simulink model "Derating_Functions"  (R2024a)
settings: Solver=VariableStepAuto  StartTime=0.0  StopTime=10.0  RelTol=1e-3
libraries: simulink x3
settings Model: Creator=ezeki  LastModifiedBy=ezeki

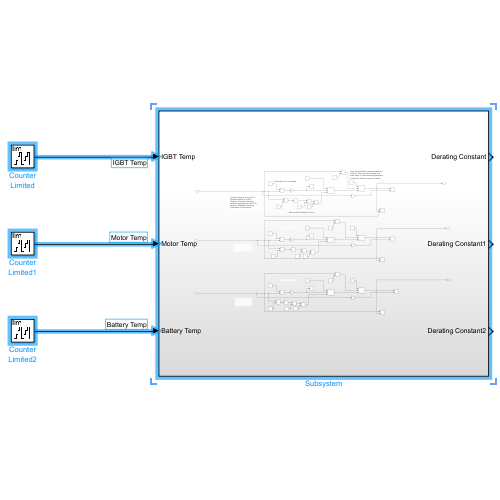
[thumbnail: Simulink's stored preview of the top-level diagram]
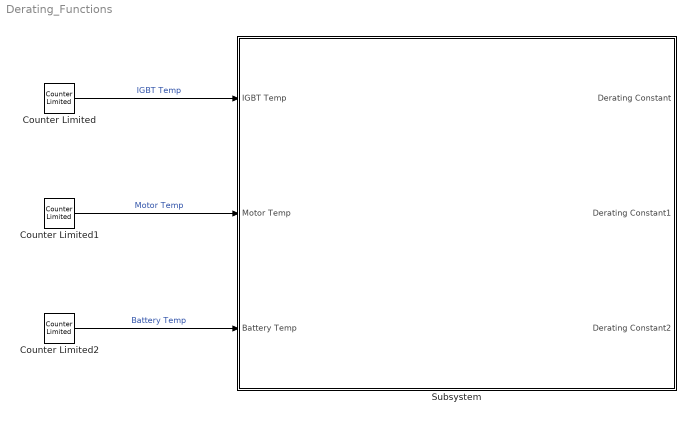
== system Derating_Functions ==
  Counter Limited : simulink/Sources/Counter Limited  uplimit=100  tsamp=0.1
  Counter Limited1 : simulink/Sources/Counter Limited  uplimit=150  tsamp=0.07
  Counter Limited2 : simulink/Sources/Counter Limited  uplimit=100  tsamp=0.1
  Subsystem : Subsystem
  wires:
  Counter Limited/1 -> Subsystem/1(IGBT Temp)  "IGBT Temp"
  Counter Limited1/1 -> Subsystem/2(Motor Temp)  "Motor Temp"
  Counter Limited2/1 -> Subsystem/3(Battery Temp)  "Battery Temp"

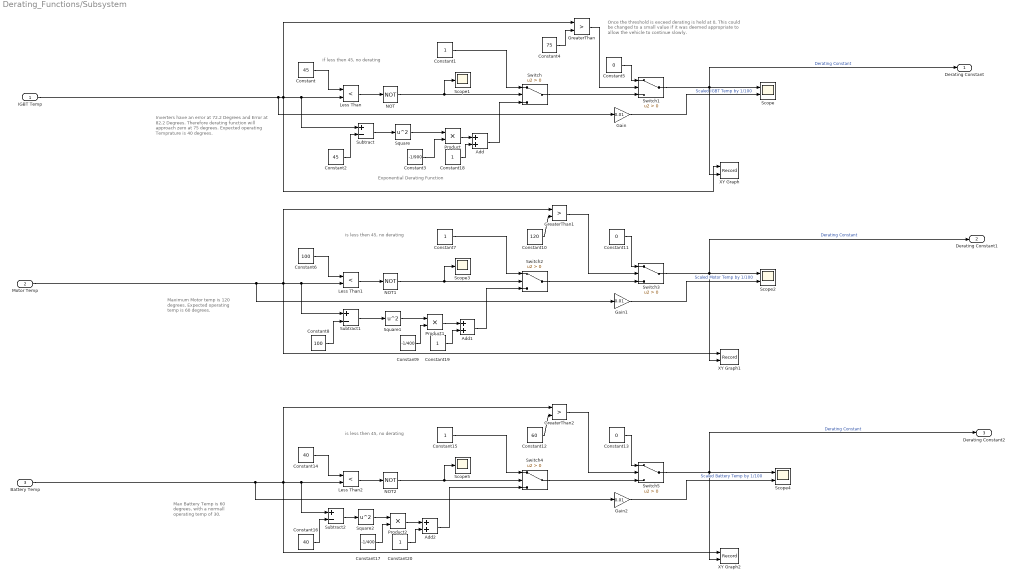
== system Derating_Functions/Subsystem ==
  note: Once the threshold is exceed derating is held at 0, This could be changed to a small value if it was deemed appropriate to allow the vehicle to continue slowly.
  note: Exponential Derating Function
  note: if less then 45, no derating
  note: Max Battery Temp is 60 degrees, with a normall operating temp of 30.
  note: Maximum Motor temp is 120 degrees. Expected operating temp is 60 degrees.
  note: Inverters have an error at 72.2 Degrees and Error at 82.2 Degrees. Therefore derating function will approach zero at 75 degrees. Expected operating Temprature is 40 degrees.
  note: is less then 45, no derating
  note: is less then 45, no derating
  IGBT Temp : Inport
  Motor Temp : Inport  Port=2
  Battery Temp : Inport  Port=3
  Add : Sum
  Add1 : Sum
  Add2 : Sum
  Constant : Constant  Value=45
  Constant{1,7,15,18..20} (6 alike) : Constant
  Constant10 : Constant  Value=120
  Constant11 : Constant  Value=0
  Constant12 : Constant  Value=60
  Constant13 : Constant  Value=0
  Constant14 : Constant  Value=40
  Constant16 : Constant  Value=40
  Constant17 : Constant  Value=-1/400
  Constant2 : Constant  Value=45
  Constant3 : Constant  Value=-1/900
  Constant4 : Constant  Value=75
  Constant5 : Constant  Value=0
  Constant6 : Constant  Value=100
  Constant8 : Constant  Value=100
  Constant9 : Constant  Value=-1/400
  Gain : Gain  Gain=0.01
  Gain1 : Gain  Gain=0.01
  Gain2 : Gain  Gain=0.01
  GreaterThan : RelationalOperator  Operator=>  OutDataTypeStr=boolean  RndMeth=Simplest  InputSameDT=off
  GreaterThan1 : RelationalOperator  Operator=>  OutDataTypeStr=boolean  RndMeth=Simplest  InputSameDT=off
  GreaterThan2 : RelationalOperator  Operator=>  OutDataTypeStr=boolean  RndMeth=Simplest  InputSameDT=off
  Less Than : RelationalOperator  Operator=<  OutDataTypeStr=boolean  RndMeth=Simplest  InputSameDT=off
  Less Than1 : RelationalOperator  Operator=<  OutDataTypeStr=boolean  RndMeth=Simplest  InputSameDT=off
  Less Than2 : RelationalOperator  Operator=<  OutDataTypeStr=boolean  RndMeth=Simplest  InputSameDT=off
  NOT : Logic  Operator=NOT  IconShape=distinctive  AllPortsSameDT=off  OutDataTypeStr=boolean
  NOT1 : Logic  Operator=NOT  IconShape=distinctive  AllPortsSameDT=off  OutDataTypeStr=boolean
  NOT2 : Logic  Operator=NOT  IconShape=distinctive  AllPortsSameDT=off  OutDataTypeStr=boolean
  Product : Product
  Product1 : Product
  Product2 : Product
  Scope : Scope  NumInputPorts=2
  Scope1 : Scope
  Scope2 : Scope  NumInputPorts=2
  Scope3 : Scope
  Scope4 : Scope  NumInputPorts=2
  Scope5 : Scope
  Square : Math  Operator=square
  Square1 : Math  Operator=square
  Square2 : Math  Operator=square
  Subtract : Sum  Inputs=+-
  Subtract1 : Sum  Inputs=+-
  Subtract2 : Sum  Inputs=+-
  Switch{,1..5} (6 alike) : Switch  Criteria=u2 > Threshold  SaturateOnIntegerOverflow=off  InputSameDT=off
  XY Graph : Record  FileSettingsInternal="{\"entries\":[{\"content\":{\"excelSettings\":{\"content\":{},\"type\":\"Streamout.ExcelSettings\"}},\"type\":\"Streamout.FileSettingStorage\",\"uuid\":\"\"}],\"packageUris\":[\"http:\\/\\/schema.mathworks.com\\/mf0\\/streamout_blocks\\/R2020a\"],\"version\":\"1.0\"}"  Layout=[1 1]  SignalsInternal="{\"entries\":[{\"content\":{\"signals\":[{\"content\":{\"blockPath\":[],\"dimensions\":[1],\"domain\":\"\",\"lineColor\":\"#a2142f\",\"plots\":[ 1 ],\"port\":1,\"signalID\":1,\"signalName\":\"IGBT Temp\"},\"type\":\"RecordBlkView.Signal\",\"uuid\":\"\"},{\"content\":{\"blockPath\":[],\"dimensions\":[1],\"domain\":\"\",\"lineColor\":\"#139fff\",\"plots\":[ 1 ],\"port\":2,\"signalID\":2,\"signalName\":\"Derating Constant\"},\"type\":\"RecordBlkView.Signal\",\"uuid\":\"\"}]},\"type\":\"RecordBlkView.InputSignals\",\"uuid\":\"\"}],\"packageUris\":[\"http:\\/\\/schema.mathworks.com\\/mf0\\/streamout_blocks\\/R2020a\"],\"version\":\"1.0\"}"  VisualizationBindings="{\"xyplotplugin\":{\"info\":[{\"series\":[{\"bindingParametersList\":[{\"parameter\":\"X-Axis\",\"signalID\":1,\"signalName\":\"IGBT Temp\"},{\"parameter\":\"Y-Axis\",\"signalID\":2,\"signalName\":\"Derating Constant\"}],\"seriesID\":0}],\"subplotID\":1}]}}"  CompatibilityTag=XY
  XY Graph1 : Record  FileSettingsInternal="{\"entries\":[{\"content\":{\"excelSettings\":{\"content\":{},\"type\":\"Streamout.ExcelSettings\"}},\"type\":\"Streamout.FileSettingStorage\",\"uuid\":\"\"}],\"packageUris\":[\"http:\\/\\/schema.mathworks.com\\/mf0\\/streamout_blocks\\/R2020a\"],\"version\":\"1.0\"}"  Layout=[1 1]  SignalsInternal="{\"entries\":[{\"content\":{\"signals\":[{\"content\":{\"blockPath\":[],\"dimensions\":[1],\"domain\":\"\",\"lineColor\":\"#a2142f\",\"plots\":[ 1 ],\"port\":1,\"signalID\":1,\"signalName\":\"Motor Temp\"},\"type\":\"RecordBlkView.Signal\",\"uuid\":\"\"},{\"content\":{\"blockPath\":[],\"dimensions\":[1],\"domain\":\"\",\"lineColor\":\"#139fff\",\"plots\":[ 1 ],\"port\":2,\"signalID\":2,\"signalName\":\"Derating Constant\"},\"type\":\"RecordBlkView.Signal\",\"uuid\":\"\"}]},\"type\":\"RecordBlkView.InputSignals\",\"uuid\":\"\"}],\"packageUris\":[\"http:\\/\\/schema.mathworks.com\\/mf0\\/streamout_blocks\\/R2020a\"],\"version\":\"1.0\"}"  VisualizationBindings="{\"xyplotplugin\":{\"info\":[{\"series\":[{\"bindingParametersList\":[{\"parameter\":\"X-Axis\",\"signalID\":1,\"signalName\":\"Motor Temp\"},{\"parameter\":\"Y-Axis\",\"signalID\":2,\"signalName\":\"Derating Constant\"}],\"seriesID\":0}],\"subplotID\":1}]}}"  CompatibilityTag=XY
  XY Graph2 : Record  FileSettingsInternal="{\"entries\":[{\"content\":{\"excelSettings\":{\"content\":{},\"type\":\"Streamout.ExcelSettings\"}},\"type\":\"Streamout.FileSettingStorage\",\"uuid\":\"\"}],\"packageUris\":[\"http:\\/\\/schema.mathworks.com\\/mf0\\/streamout_blocks\\/R2020a\"],\"version\":\"1.0\"}"  Layout=[1 1]  SignalsInternal="{\"entries\":[{\"content\":{\"signals\":[{\"content\":{\"blockPath\":[],\"dimensions\":[1],\"domain\":\"\",\"lineColor\":\"#a2142f\",\"plots\":[ 1 ],\"port\":1,\"signalID\":1,\"signalName\":\"Battery Temp\"},\"type\":\"RecordBlkView.Signal\",\"uuid\":\"\"},{\"content\":{\"blockPath\":[],\"dimensions\":[1],\"domain\":\"\",\"lineColor\":\"#139fff\",\"plots\":[ 1 ],\"port\":2,\"signalID\":2,\"signalName\":\"Derating Constant\"},\"type\":\"RecordBlkView.Signal\",\"uuid\":\"\"}]},\"type\":\"RecordBlkView.InputSignals\",\"uuid\":\"\"}],\"packageUris\":[\"http:\\/\\/schema.mathworks.com\\/mf0\\/streamout_blocks\\/R2020a\"],\"version\":\"1.0\"}"  VisualizationBindings="{\"xyplotplugin\":{\"info\":[{\"series\":[{\"bindingParametersList\":[{\"parameter\":\"X-Axis\",\"signalID\":1,\"signalName\":\"Battery Temp\"},{\"parameter\":\"Y-Axis\",\"signalID\":2,\"signalName\":\"Derating Constant\"}],\"seriesID\":0}],\"subplotID\":1}]}}"  CompatibilityTag=XY
  Derating Constant : Outport
  Derating Constant1 : Outport  Port=2
  Derating Constant2 : Outport  Port=3
  wires:
  Add/1 -> Switch/3
  Less Than2/1 -> NOT2/1
  Motor Temp/1 -> XY Graph1/1, GreaterThan1/1, Subtract1/1, Less Than1/2, Gain1/1
  NOT2/1 -> Scope5/1, Switch4/2
  Constant7/1 -> Switch2/1
  Switch1/1 -> Derating Constant/1, Scope/1, XY Graph/2  "Derating Constant"
  Gain1/1 -> Scope2/2  "Scaled Motor Temp by 1/100"
  NOT1/1 -> Scope3/1, Switch2/2
  GreaterThan/1 -> Switch1/2
  Constant18/1 -> Add/2
  Constant16/1 -> Subtract2/2
  Subtract1/1 -> Square1/1
  Constant1/1 -> Switch/1
  Battery Temp/1 -> XY Graph2/1, GreaterThan2/1, Subtract2/1, Less Than2/2, Gain2/1
  Subtract2/1 -> Square2/1
  Constant5/1 -> Switch1/1
  Switch/1 -> Switch1/3
  Less Than/1 -> NOT/1
  Product1/1 -> Add1/1
  Constant2/1 -> Subtract/2
  Constant6/1 -> Less Than1/1
  Subtract/1 -> Square/1
  Gain2/1 -> Scope4/2  "Scaled Battery Temp by 1/100"
  Add1/1 -> Switch2/3
  Add2/1 -> Switch4/3
  Constant19/1 -> Add1/2
  Constant8/1 -> Subtract1/2
  Square/1 -> Product/1
  Constant9/1 -> Product1/2
  Constant4/1 -> GreaterThan/2
  IGBT Temp/1 -> Gain/1, XY Graph/1, GreaterThan/1, Subtract/1, Less Than/2
  Constant10/1 -> GreaterThan1/2
  Gain/1 -> Scope/2  "Scaled IGBT Temp by 1/100"
  Switch2/1 -> Switch3/3
  Switch3/1 -> Derating Constant1/1, Scope2/1, XY Graph1/2  "Derating Constant"
  Constant3/1 -> Product/2
  Constant14/1 -> Less Than2/1
  Constant20/1 -> Add2/2
  Switch4/1 -> Switch5/3
  Square1/1 -> Product1/1
  Less Than1/1 -> NOT1/1
  Constant11/1 -> Switch3/1
  Constant12/1 -> GreaterThan2/2
  Square2/1 -> Product2/1
  GreaterThan1/1 -> Switch3/2
  Switch5/1 -> Derating Constant2/1, Scope4/1, XY Graph2/2  "Derating Constant"
  Constant13/1 -> Switch5/1
  Product/1 -> Add/1
  Constant/1 -> Less Than/1
  Constant15/1 -> Switch4/1
  NOT/1 -> Scope1/1, Switch/2
  Product2/1 -> Add2/1
  Constant17/1 -> Product2/2
  GreaterThan2/1 -> Switch5/2
